simulink model "dwupolozeniowy"  (R2018b)
settings: Solver=VariableStepAuto  StartTime=0.0  StopTime=100  RelTol=1e-3
settings Model: Creator=groinder  LastModifiedBy=groinder

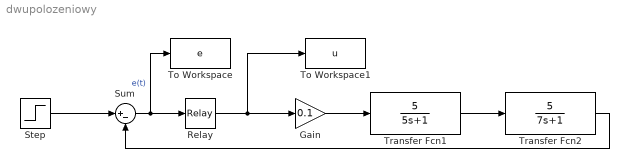
== system dwupolozeniowy ==
  Gain : Gain  Gain=0.1
  Relay : Relay  OnSwitchValue=0.8  OffSwitchValue=-0.8
  Step : Step  SampleTime=0
  Sum : Sum  Inputs=|+-
  To Workspace : ToWorkspace  VariableName=e  SaveFormat=Structure With Time  SampleTime=-1
  To Workspace1 : ToWorkspace  VariableName=u  SaveFormat=Structure With Time  SampleTime=-1
  Transfer Fcn1 : TransferFcn  Numerator=[5]  Denominator=[5 1]
  Transfer Fcn2 : TransferFcn  Numerator=[5]  Denominator=[7 1]
  wires:
  Step/1 -> Sum/1
  Sum/1 -> To Workspace/1, Relay/1  "e(t)"
  Relay/1 -> Gain/1, To Workspace1/1
  Transfer Fcn1/1 -> Transfer Fcn2/1
  Transfer Fcn2/1 -> Sum/2
  Gain/1 -> Transfer Fcn1/1
